simulink model "PIDControl_1DoFSim"  (R2023b)
settings: Solver=VariableStepAuto  StartTime=0.0  StopTime=4  RelTol=1e-3
values from neighbouring files (symbols this model uses):
  desiredBodyRates = [0 0 0]    [init_1DoFSim.m]
  Inertia = [ .10 0 0 ... (first row only)    [init_1DoFSim.m]
  kd = -3    [init_1DoFSim.m]
  ki = -.5    (= -0.5)    [init_1DoFSim.m]
  kp = -10    [init_1DoFSim.m]
  Moments = [0 0 0]    [init_1DoFSim.m]
  P_pulse = .1    (= 0.1)    [init_1DoFSim.m]
  pqr_0 = [0 0 0]'    [init_1DoFSim.m]
  q_0 = Euler_To_Quaternion_ScalarFirst(Euler_Initial)'    [init_1DoFSim.m]
  q_desired = Euler_To_Quaternion_ScalarFirst(Euler_Desired)'    [init_1DoFSim.m]
  Thrust_Moment = 14.2    [init_1DoFSim.m]
libraries: aerolibanimutils x1, matrix_library x1, aerolibutil x1, vrlib x1
settings Model: Creator=benjackson  LastModifiedBy=ben
settings OptimizationCC: ReuseModelBlockBuffer=off

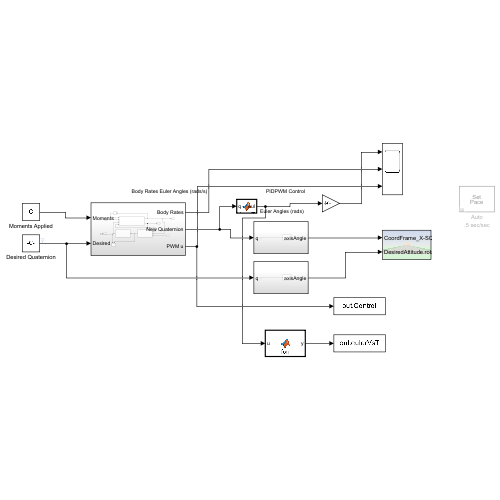
[thumbnail: Simulink's stored preview of the top-level diagram]
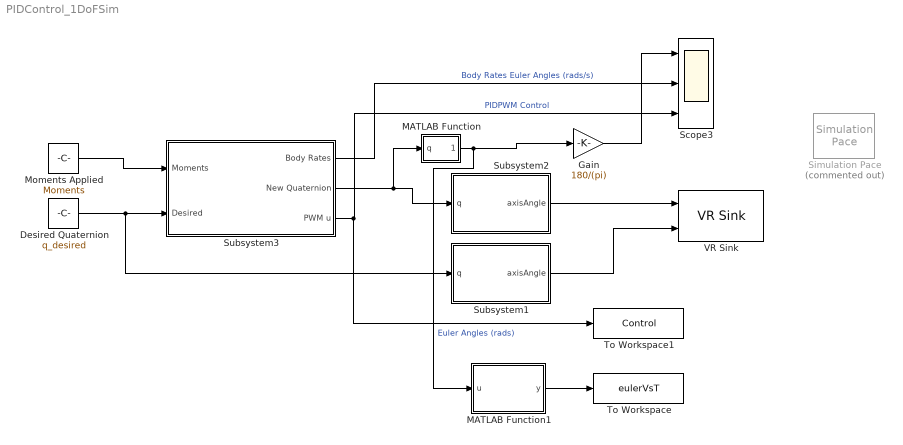
== system PIDControl_1DoFSim ==
  Desired Quaternion : Constant  Value=q_desired
  Gain : Gain  Gain=180/(pi)
  MATLAB Function : MATLAB Function  TreatAsAtomicUnit=on
  MATLAB Function1 : MATLAB Function  TreatAsAtomicUnit=on
  Moments Applied : Constant  Value=Moments
  Scope3 : Scope  NumInputPorts=3
  Simulation Pace : aerolibanimutils/Simulation Pace  Commented=on  SimulationPace=.5  SleepMode=Auto  OutputPaceError=off  SampleTime=1/30
  Subsystem1 : Subsystem
  Subsystem2 : Subsystem
  Subsystem3 : Subsystem
  To Workspace : ToWorkspace  VariableName=eulerVsT  SaveFormat=Timeseries  SampleTime=-1
  To Workspace1 : ToWorkspace  VariableName=Control  SaveFormat=Timeseries  SampleTime=-1
  VR Sink : vrlib/VR Sink  InstantiateOnLoad=on  SampleTime=0.1  ViewEnable=on  RemoteChange=off  RemoteView=off  FieldsWritten=CoordFrame_X-SQUARE_Y-CIRCLE_Z-OCTOGO_Transform.rotation.4.1.1.double#DesiredAttitude.rotation.4.1.1.double  WorldFileName=World/World_RXN_WHL.x3d  WorldDescription=Straight Road Strip - 2 Lanes  AutoView=off  VideoDimensions=[]  AllowVariableSize=off
  wires:
  Moments Applied/1 -> Subsystem3/1(Moments)
  Subsystem3/1(Body Rates) -> Scope3/2  "Body Rates Euler Angles (rads/s)"
  Subsystem2/1(axisAngle) -> VR Sink/1
  Desired Quaternion/1 -> Subsystem1/1(q), Subsystem3/2(Desired)
  Subsystem1/1(axisAngle) -> VR Sink/2
  MATLAB Function/1(eul) -> MATLAB Function1/1(u), Gain/1  "Euler Angles (rads)"
  Subsystem3/3(PWM u) -> To Workspace1/1, Scope3/3  "PIDPWM Control"
  Gain/1 -> Scope3/1
  MATLAB Function1/1(y) -> To Workspace/1
  Subsystem3/2(New Quaternion) -> Subsystem2/1(q), MATLAB Function/1(q)

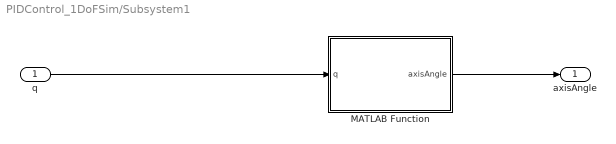
== system PIDControl_1DoFSim/Subsystem1 ==
  q : Inport
  MATLAB Function : MATLAB Function  TreatAsAtomicUnit=on
  axisAngle : Outport
  wires:
  q/1 -> MATLAB Function/1(q)
  MATLAB Function/1(axisAngle) -> axisAngle/1

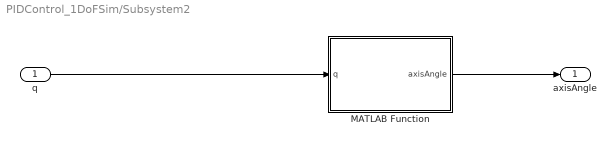
== system PIDControl_1DoFSim/Subsystem2 ==
  q : Inport
  MATLAB Function : MATLAB Function  TreatAsAtomicUnit=on
  axisAngle : Outport
  wires:
  q/1 -> MATLAB Function/1(q)
  MATLAB Function/1(axisAngle) -> axisAngle/1

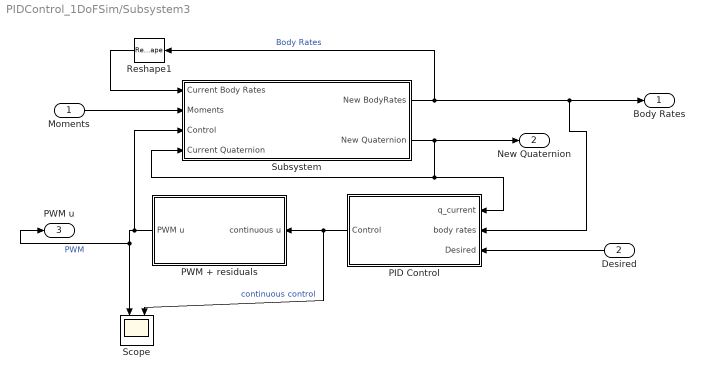
== system PIDControl_1DoFSim/Subsystem3 ==
  Moments : Inport
  Desired : Inport  Port=2
  PID Control : Subsystem
  PWM + residuals : Subsystem
  Reshape1 : Reshape  OutputDimensionality=Customize  OutputDimensions=[1,3]
  Scope : Scope  NumInputPorts=2
  Subsystem : Subsystem
  Body Rates : Outport
  New Quaternion : Outport  Port=2
  PWM u : Outport  Port=3
  wires:
  Subsystem/1(New BodyRates) -> Reshape1/1, PID Control/2(body rates), Body Rates/1  "Body Rates"
  Subsystem/2(New Quaternion) -> New Quaternion/1, PID Control/1(q_current), Subsystem/4(Current Quaternion)
  Reshape1/1 -> Subsystem/1(Current Body Rates)
  Desired/1 -> PID Control/3(Desired)
  Moments/1 -> Subsystem/2(Moments)
  PID Control/1(Control) -> Scope/2, PWM + residuals/1(continuous u)  "continuous control"
  PWM + residuals/1(PWM u) -> Subsystem/3(Control), PWM u/1, Scope/1  "PWM"

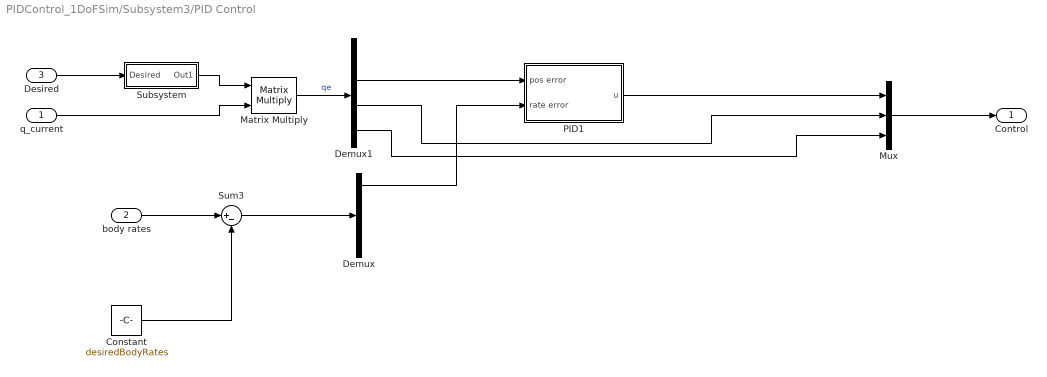
== system PIDControl_1DoFSim/Subsystem3/PID Control ==
  q_current : Inport
  body rates : Inport  Port=2
  Desired : Inport  Port=3
  Constant : Constant  Value=desiredBodyRates
  Demux : Demux  Outputs=3
  Demux1 : Demux
  Matrix Multiply : Product  Multiplication=Matrix(*)
  Mux : Mux  Inputs=3
  PID1 : Subsystem
  Subsystem : Subsystem
  Sum3 : Sum  Inputs=|+-
  Control : Outport
  wires:
  Desired/1 -> Subsystem/1(Desired)
  Subsystem/1(Out1) -> Matrix Multiply/1
  q_current/1 -> Matrix Multiply/2
  body rates/1 -> Sum3/1
  Matrix Multiply/1 -> Demux1/1  "qe"
  Demux/1 -> PID1/2(rate error)
  Demux1/2 -> PID1/1(pos error)
  Mux/1 -> Control/1
  Demux1/3 -> Mux/2
  Demux1/4 -> Mux/3
  PID1/1(u) -> Mux/1
  Sum3/1 -> Demux/1
  Constant/1 -> Sum3/2

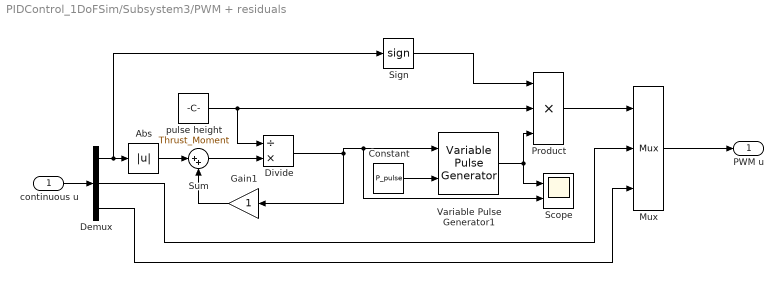
== system PIDControl_1DoFSim/Subsystem3/PWM + residuals ==
  continuous u : Inport
  Abs : Abs  SaturateOnIntegerOverflow=off
  Constant : Constant  Value=P_pulse
  Demux : Demux  Outputs=3
  Divide : Product  Inputs=/*
  Gain1 : Gain
  Mux : Mux  Inputs=3
  Product : Product  Inputs=3
  Scope : Scope  NumInputPorts=2
  Sign : Signum
  Sum : Sum  Inputs=|++
  Variable Pulse Generator1 : VariablePulseGenerator  AllowZeroPulseWidth=on  SampleTime=0.1
  pulse height : Constant  Value=Thrust_Moment
  PWM u : Outport
  wires:
  continuous u/1 -> Demux/1
  Divide/1 -> Variable Pulse Generator1/1, Scope/2, Gain1/1
  Gain1/1 -> Sum/2
  Sum/1 -> Divide/2
  Product/1 -> Mux/1
  pulse height/1 -> Product/2, Divide/1
  Variable Pulse Generator1/1 -> Product/3, Scope/1
  Constant/1 -> Variable Pulse Generator1/2
  Demux/2 -> Mux/2
  Demux/3 -> Mux/3
  Mux/1 -> PWM u/1
  Demux/1 -> Sign/1, Abs/1
  Abs/1 -> Sum/1
  Sign/1 -> Product/1

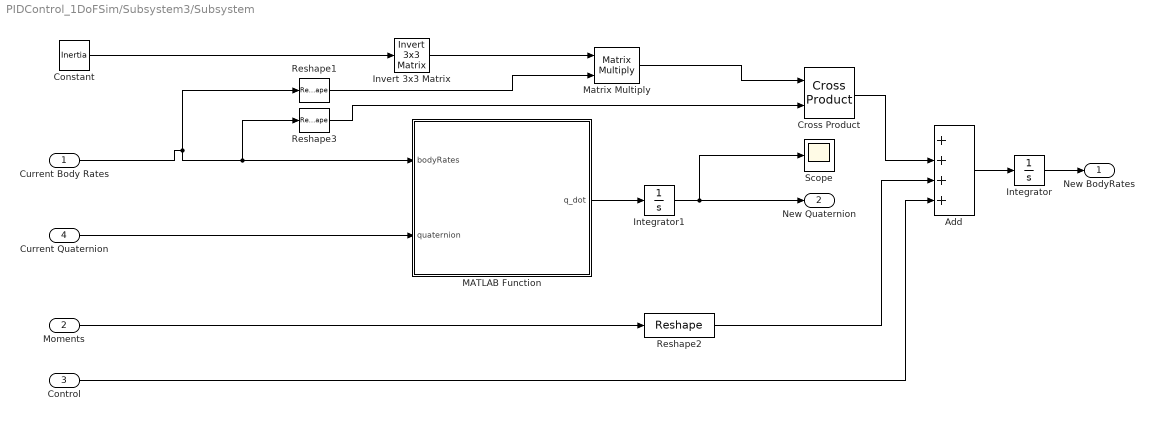
== system PIDControl_1DoFSim/Subsystem3/Subsystem ==
  Current Body Rates : Inport
  Moments : Inport  Port=2
  Control : Inport  Port=3
  Current Quaternion : Inport  Port=4
  Add : Sum  Inputs=++++
  Constant : Constant  Value=Inertia
  Cross Product : matrix_library/Cross Product
  Integrator : Integrator  InitialCondition=pqr_0
  Integrator1 : Integrator  InitialCondition=q_0
  Invert 3x3 Matrix : aerolibutil/Invert  3x3 Matrix
  MATLAB Function : MATLAB Function  TreatAsAtomicUnit=on
  Matrix Multiply : Product  Multiplication=Matrix(*)
  Reshape1 : Reshape  OutputDimensionality=Customize  OutputDimensions=[3,1]
  Reshape2 : Reshape  OutputDimensionality=Customize  OutputDimensions=[3,1]
  Reshape3 : Reshape  OutputDimensionality=Customize  OutputDimensions=[3,1]
  Scope : Scope
  New BodyRates : Outport
  New Quaternion : Outport  Port=2
  wires:
  Matrix Multiply/1 -> Cross Product/1
  Current Quaternion/1 -> MATLAB Function/2(quaternion)
  Constant/1 -> Invert 3x3 Matrix/1
  MATLAB Function/1(q_dot) -> Integrator1/1
  Current Body Rates/1 -> Reshape1/1, Reshape3/1, MATLAB Function/1(bodyRates)
  Invert 3x3 Matrix/1 -> Matrix Multiply/1
  Cross Product/1 -> Add/2
  Add/1 -> Integrator/1
  Moments/1 -> Reshape2/1
  Reshape3/1 -> Cross Product/2
  Reshape1/1 -> Matrix Multiply/2
  Reshape2/1 -> Add/3
  Integrator1/1 -> Scope/1, New Quaternion/1
  Control/1 -> Add/4
  Integrator/1 -> New BodyRates/1

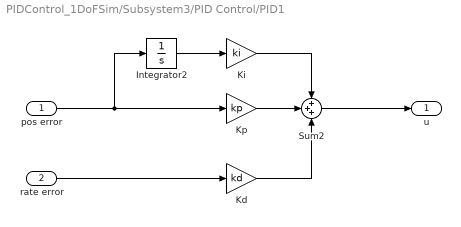
== system PIDControl_1DoFSim/Subsystem3/PID Control/PID1 ==
  pos error : Inport
  rate error : Inport  Port=2
  Integrator2 : Integrator
  Kd : Gain  Gain=kd
  Ki : Gain  Gain=ki
  Kp : Gain  Gain=kp
  Sum2 : Sum  Inputs=+++
  u : Outport
  wires:
  Sum2/1 -> u/1
  rate error/1 -> Kd/1
  Ki/1 -> Sum2/1
  pos error/1 -> Integrator2/1, Kp/1
  Integrator2/1 -> Ki/1
  Kd/1 -> Sum2/3
  Kp/1 -> Sum2/2

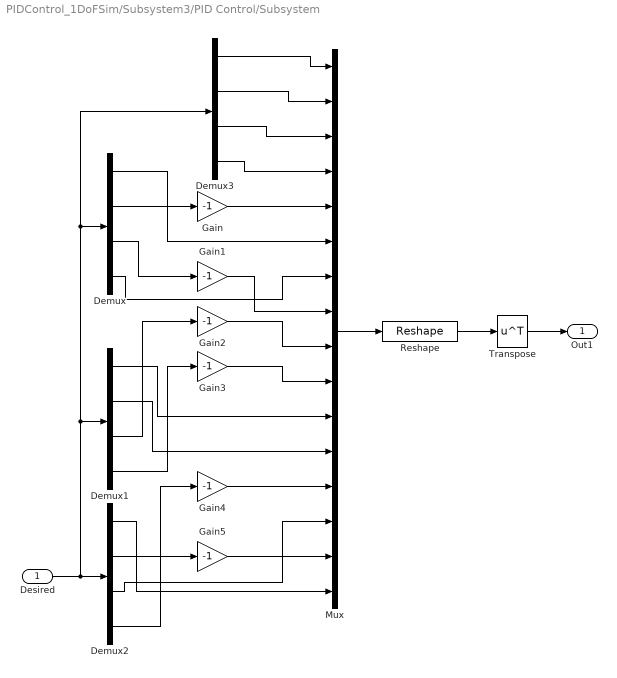
== system PIDControl_1DoFSim/Subsystem3/PID Control/Subsystem ==
  Desired : Inport
  Demux{,1..3} (4 alike) : Demux
  Gain{,1..5} (6 alike) : Gain  Gain=-1
  Mux : Mux  Inputs=16
  Reshape : Reshape  OutputDimensionality=Customize  OutputDimensions=[4,4]
  Transpose : Math  Operator=transpose
  Out1 : Outport
  wires:
  Reshape/1 -> Transpose/1
  Mux/1 -> Reshape/1
  Gain5/1 -> Mux/15
  Demux3/3 -> Mux/3
  Gain2/1 -> Mux/9
  Gain1/1 -> Mux/8
  Demux3/4 -> Mux/4
  Demux3/2 -> Mux/2
  Demux3/1 -> Mux/1
  Demux2/4 -> Gain4/1
  Demux2/3 -> Mux/14
  Demux1/4 -> Gain3/1
  Demux/2 -> Gain/1
  Demux1/3 -> Gain2/1
  Demux/3 -> Gain1/1
  Transpose/1 -> Out1/1
  Demux2/2 -> Gain5/1
  Demux1/1 -> Mux/11
  Demux1/2 -> Mux/12
  Demux/4 -> Mux/7
  Gain4/1 -> Mux/13
  Demux2/1 -> Mux/16
  Gain3/1 -> Mux/10
  Demux/1 -> Mux/6
  Gain/1 -> Mux/5
  Desired/1 -> Demux/1, Demux3/1, Demux1/1, Demux2/1

== matlab function PIDControl_1DoFSim/MATLAB Function1 ==
  data: u input; y output
function y = fcn(u)
    
y = u(1);

== matlab function PIDControl_1DoFSim/MATLAB Function ==
  data: q input; eul output
function eul = Quaternion_To_Euler(q)
   
    qw = q(4);
    qx = q(1);
    qy = q(2);
    qz = q(3);
    q_mag = qw^2 +qx^2 +qy^2 +qz^2;
    
    q = q./q_mag;
    
    % Pre-allocate output
    eul = zeros(1, 3, 'like', q);
    
    % Cap all inputs to asin to 1, since values >1 produce complex
    % results
    % Since the quaternion is of unit length, this should never happen,
    % but some code generation configuration seem to hit this edge case
    % under some circumstances.
    aSinInput = -2*(qx.*qz-qw.*qy);
    mask1 = aSinInput >= 1 - 10*eps(class(qw));
    mask2 = aSinInput <= -1 + 10*eps(class(qw));
    aSinInput(mask1) = 1;
    aSinInput(mask2) = -1 ;
    mask = mask1 | mask2;
    
    eul = [ atan2( 2*(qx.*qy+qw.*qz), qw.^2 + qx.^2 - qy.^2 - qz.^2 ), ...
        asin( aSinInput ), ...
        atan2( 2*(qy.*qz+qw.*qx), qw.^2 - qx.^2 - qy.^2 + qz.^2 )];
    eul(mask, 1) = -sign(aSinInput(mask,1)).* 2 .* atan2(qx(mask,1), qw(mask,1));
    eul(mask, 3) = 0;
    
    % Check for complex numbers
    if ~isreal(eul)
        eul = real(eul);
    end
    
%     if nargout > 1
%         eul; % workaround for g2380983 (const folding heurstic issue during codegen)
%         eulAlt = robotics.core.internal.generateAlternateEulerAngles(eul, seq);
%     end
    
    
end

== matlab function PIDControl_1DoFSim/Subsystem2/MATLAB Function ==
  data: q input; axisAngle output

function axisAngle = Quaternion_To_AxisAngle(q)
    for  i = 1:4
        if q(i) > 1 
            q(i) = 1.0;
            disp(q)
        end
    end

    qw = q(1);
    qx = q(2);
    qy = q(3);
    qz = q(4);
  

    theta = 2*acos(qw);

    if theta == 0 
        x = 1;
        y = 0;
        z = 0;
    else
        x = qx/(sin(theta/2));
        y = qy/(sin(theta/2));
        z = qz/(sin(theta/2));
    end
    
    %Vector comes first in our axis representation and angle comes last
    axisAngle = [x,z,y,theta];

end

== matlab function PIDControl_1DoFSim/Subsystem3/Subsystem/MATLAB Function ==
  data: bodyRates input; quaternion input; q_dot output
function q_dot = getBodyRates(bodyRates,quaternion)

    p = bodyRates(1);
    q = bodyRates(2); 
    r = bodyRates(3);
    
    half_Q_Matrix =   0.5 * [  0, -p, -q, -r
                               p,  0,  r, -q
                               q, -r,  0,  p
                               r,  q, -p,  0];
                
    qVec  =  [quaternion(1); quaternion(2); quaternion(3); quaternion(4)];
    q_dot =  (half_Q_Matrix * qVec);     
    
end

== matlab function PIDControl_1DoFSim/Subsystem1/MATLAB Function ==
  data: q input; axisAngle output

function axisAngle = Quaternion_To_AxisAngle(q)
    for  i = 1:4
        if q(i) > 1 
            q(i) = 1.0;
            disp(q)
        end
    end

    qw = q(1);
    qx = q(2);
    qy = q(3);
    qz = q(4);
  

    theta = 2*acos(qw);

    if theta == 0 
        x = 1;
        y = 0;
        z = 0;
    else
        x = qx/(sin(theta/2));
        y = qy/(sin(theta/2));
        z = qz/(sin(theta/2));
    end
    
    %Vector comes first in our axis representation and angle comes last
    axisAngle = [x,z,y,theta];

end
